simulink model "blockdemo"  (Simulink 6.3)
settings: Solver=FixedStepDiscrete  StartTime=0  StopTime=100  FixedStep=1  RelTol=1e-3
InitFcn:
  | %% DSPBuilder Start
  | alt_dspbuilder_update_model(bdroot)
  | %% DSPBuilder End
libraries: allblocks_alteradspbuilder2 x14, simulink x1
settings Model: Creator=mjervis  LastModifiedBy=delphick
settings OptimizationCC: BooleanDataType=off  InlineInvariantSignals=on
settings DebuggingCC: SolverPrmCheckMsg=none
settings HardwareCC: TargetUnknown=on

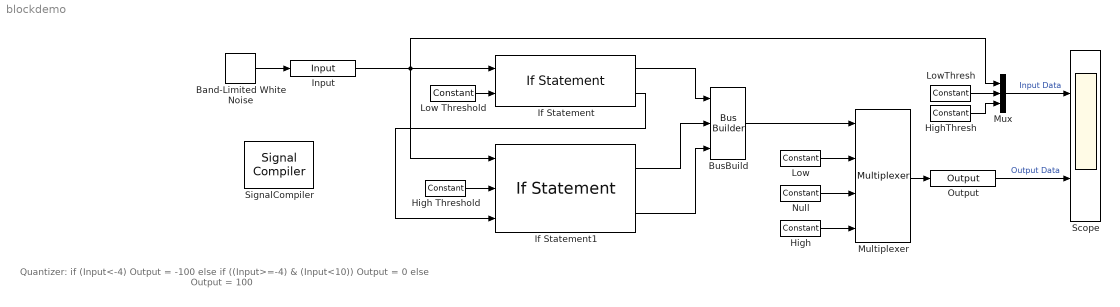
== system blockdemo ==
  note: Quantizer:
      | if (Input<-4)  Output = -100
      | else if ((Input>=-4) & (Input<10)) Output = 0
      | else Output = 100
  Band-Limited White Noise : simulink/Sources/Band-Limited White Noise  Cov=[126]  Ts=1  seed=[23341]
  BusBuild : allblocks_alteradspbuilder2/Bus Builder  BusType=Unsigned Integer  bwl=3  bwr=0
  High : allblocks_alteradspbuilder2/Constant  mask_cst=100  BusType=Signed Integer  bwl=8  bwr=0  SpecifyClock=off
  High Threshold : allblocks_alteradspbuilder2/Constant  mask_cst=10  BusType=Signed Integer  bwl=8  bwr=0  SpecifyClock=off
  HighThresh : allblocks_alteradspbuilder2/Constant  mask_cst=10  BusType=Signed Integer  bwl=8  bwr=0  SpecifyClock=off
  If Statement : allblocks_alteradspbuilder2/If Statement  user_inputs=2  if_expression=a<b  BusType=Inferred  bwl=8  bwr=0  use_else_output=on  use_elseif_input=off
  If Statement1 : allblocks_alteradspbuilder2/If Statement  user_inputs=2  if_expression=a<b  BusType=Inferred  bwl=8  bwr=0  use_else_output=on  use_elseif_input=on
  Input : allblocks_alteradspbuilder2/Input  iofile=C:\workspace_clean\Documentation\DesignExamples\Tutorials\UnitBlocks\GateAndControl\IfStatement\tb_blockdemo\blockdemo_Input.salt  BusType=Signed Integer  bwl=8  bwr=0  SpecifyClock=off  PORTTYPE=Input
  Low : allblocks_alteradspbuilder2/Constant  mask_cst=-100  BusType=Signed Integer  bwl=8  bwr=0  SpecifyClock=off
  Low Threshold : allblocks_alteradspbuilder2/Constant  mask_cst=-4  BusType=Signed Integer  bwl=8  bwr=0  SpecifyClock=off
  LowThresh : allblocks_alteradspbuilder2/Constant  mask_cst=-4  BusType=Signed Integer  bwl=8  bwr=0  SpecifyClock=off
  Multiplexer : allblocks_alteradspbuilder2/Multiplexer  numInputs=3  pipeline=0  oneHot=on  use_ena=off  use_aclr=off
  Mux : Mux  Inputs=3
  Null : allblocks_alteradspbuilder2/Constant  mask_cst=0  BusType=Signed Integer  bwl=8  bwr=0  SpecifyClock=off
  Output : allblocks_alteradspbuilder2/Output  iofile=C:\workspace_clean\Documentation\DesignExamples\Tutorials\UnitBlocks\GateAndControl\IfStatement\tb_blockdemo\blockdemo_Output.capture  BusType=Signed Integer  bwl=8  bwr=0  PORTTYPE=Output
  Scope : Scope  NumInputPorts=2
      settings: YMin=-40~-120  YMax=40~120
  SignalCompiler : allblocks_alteradspbuilder2/Signal Compiler  DeviceFamily=Stratix IV  DeviceName=AUTO  EnableSignalTap=off  SignalTapDepth=128  UseBoardBlock=off  StpUseDefaultClock=on  StpClock=clock
  wires:
  Low Threshold/1 -> If Statement/2
  Input/1 -> If Statement/1, If Statement1/1, Mux/1
  High Threshold/1 -> If Statement1/2
  Band-Limited White Noise/1 -> Input/1
  Output/1 -> Scope/2  "Output Data"
  If Statement/2 -> If Statement1/3
  If Statement/1 -> BusBuild/1
  If Statement1/1 -> BusBuild/2
  If Statement1/2 -> BusBuild/3
  LowThresh/1 -> Mux/2
  HighThresh/1 -> Mux/3
  Mux/1 -> Scope/1  "Input Data"
  BusBuild/1 -> Multiplexer/1
  Low/1 -> Multiplexer/2
  Null/1 -> Multiplexer/3
  High/1 -> Multiplexer/4
  Multiplexer/1 -> Output/1
